simulink library "gm_TxLUT_RxCapture_4x4_HDL_IQ_lib"  (R2019b)
settings: Solver=VariableStepAuto  StartTime=0.0  StopTime=10.0  RelTol=1e-3
undefined symbols (not defined in the file or in its folder): AXI4, Lite
libraries: axiinterfacelib x11
settings Model: Creator=ajtro  LastModifiedBy=ajtro

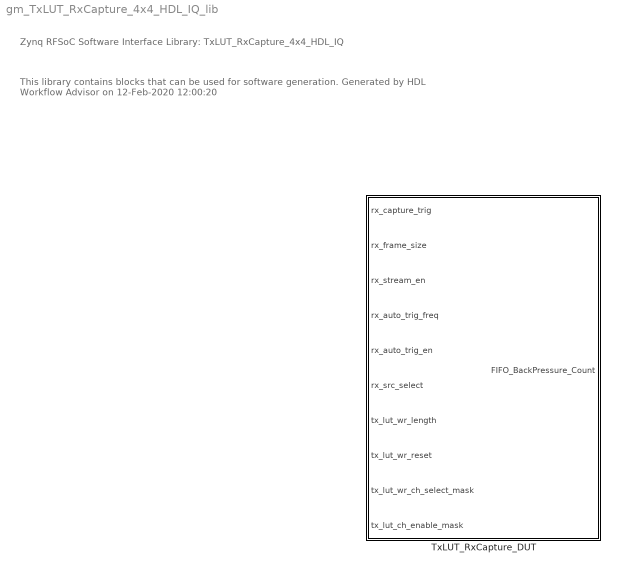
== system gm_TxLUT_RxCapture_4x4_HDL_IQ_lib ==
  note: Zynq RFSoC Software Interface Library: TxLUT_RxCapture_4x4_HDL_IQ
  note: This library contains blocks that can be used for software generation.
      |
      | Generated by HDL Workflow Advisor on 12-Feb-2020 12:00:20
  TxLUT_RxCapture_DUT : Subsystem  TreatAsAtomicUnit=on  mask(AXI4-Lite/AXI4 Interface){}
      mask help:
      | This is an automatically generated subsystem block.
      | This contains the AXI interface blocks that communicate with the DAC_ADC_HDL_Coder_IP IPCore generated from TxLUT_RxCapture_4x4_HDL_IQ/TxLUT_RxCapture_DUT subsystem.
      mask Display: disp(sprintf('Xilinx Zynq \nAXI Interface'));

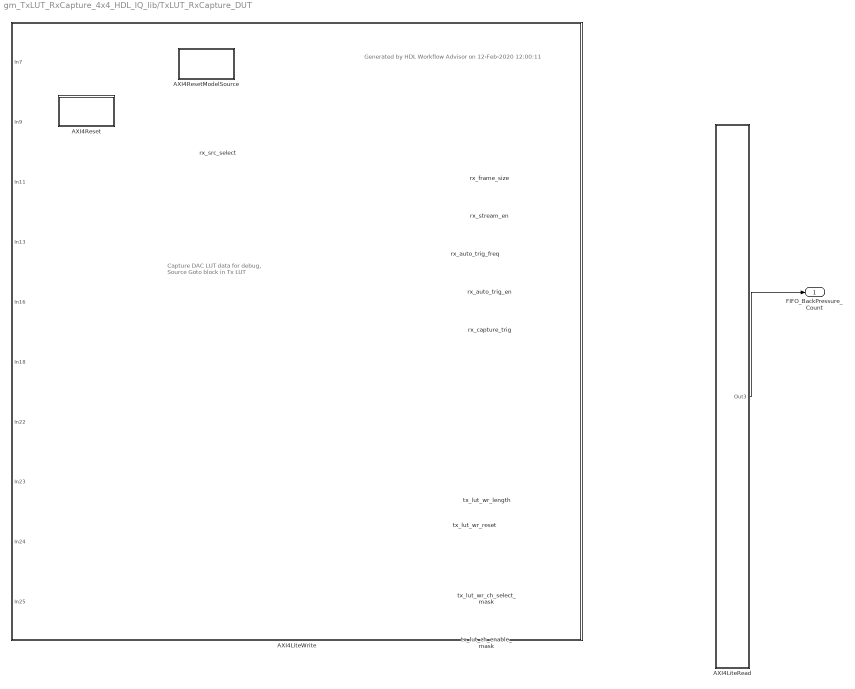
== system gm_TxLUT_RxCapture_4x4_HDL_IQ_lib/TxLUT_RxCapture_DUT ==
  note: Generated by HDL Workflow Advisor on 12-Feb-2020 12:00:11
  note: Capture DAC LUT data for debug,
      | Source Goto block in Tx LUT
  rx_capture_trig : Inport
  rx_frame_size : Inport  Port=2
  rx_stream_en : Inport  Port=3
  rx_auto_trig_freq : Inport  Port=4
  rx_auto_trig_en : Inport  Port=5
  rx_src_select : Inport  Port=6  OutDataTypeStr=fixdt(0,1,0)
  tx_lut_wr_length : Inport  Port=7
  tx_lut_wr_reset : Inport  Port=8
  tx_lut_wr_ch_select_mask : Inport  Port=9
  tx_lut_ch_enable_mask : Inport  Port=10
  AXI4LiteRead : Subsystem  Priority=10
  AXI4LiteWrite : Subsystem  Priority=1
  AXI4Reset : Subsystem  mask(System Start){ShowInLibBrowser=0}
      mask prompts: ShowInLibBrowser "Simulink:masks:CustCodeMaskParam1_MP"
      settings: CopyFcn=cccopyfcn(gcb)  OpenFcn=ccopenfcn('System Start Function')
      mask Help: eval('feval(''rtwprivate'',''rtwhelpview'',''rtw_sys_start_block'')');
      mask Display: disp('System\nStart');
  AXI4ResetModelSource : Subsystem  mask(Model Source){ShowInLibBrowser=0}
      mask prompts: ShowInLibBrowser "Simulink:masks:CustCodeMaskParam1_MP"
      settings: CopyFcn=cccopyfcn(gcb)  OpenFcn=ccopenfcn('Model Source')
      mask Help: eval('feval(''rtwprivate'',''rtwhelpview'',''rtw_model_source_block'')');
      mask Display: disp('Model\nSource');
  FIFO_BackPressure_Count : Outport  VectorParamsAs1DForOutWhenUnconnected=off
  wires:
  AXI4LiteRead/1(Out3) -> FIFO_BackPressure_Count/1
  tx_lut_ch_enable_mask/1 -> AXI4LiteWrite/10(In25)
  tx_lut_wr_ch_select_mask/1 -> AXI4LiteWrite/9(In24)
  tx_lut_wr_reset/1 -> AXI4LiteWrite/8(In23)
  tx_lut_wr_length/1 -> AXI4LiteWrite/7(In22)
  rx_capture_trig/1 -> AXI4LiteWrite/6(In18)
  rx_auto_trig_en/1 -> AXI4LiteWrite/5(In16)
  rx_auto_trig_freq/1 -> AXI4LiteWrite/4(In13)
  rx_stream_en/1 -> AXI4LiteWrite/3(In11)
  rx_frame_size/1 -> AXI4LiteWrite/2(In9)
  rx_src_select/1 -> AXI4LiteWrite/1(In7)

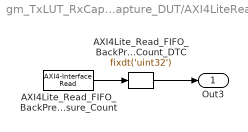
== system gm_TxLUT_RxCapture_4x4_HDL_IQ_lib/TxLUT_RxCapture_DUT/AXI4LiteRead ==
  AXI4Lite_Read_FIFO_BackPressure_Count : axiinterfacelib/AXI4-Interface Read  Priority=5  AXIInterfaceType=AXI4-Lite  DeviceName=/dev/mwipcore  RegisterOffset=hex2dec('134')  DataLength=1  DataType=uint32  SampleTime=-1  blockPlatform=ZYNQ  SimulateUsing=Interpreted Execution
      settings: SourceProductName=Embedded Coder Support Package for Xilinx Zynq Platform  SourceProductBaseCode=ECZYNQ7000
  AXI4Lite_Read_FIFO_BackPressure_Count_DTC : DataTypeConversion  OutDataTypeStr=fixdt('uint32')  ConvertRealWorld=Stored Integer (SI)
  Out3 : Outport
  wires:
  AXI4Lite_Read_FIFO_BackPressure_Count_DTC/1 -> Out3/1
  AXI4Lite_Read_FIFO_BackPressure_Count/1 -> AXI4Lite_Read_FIFO_BackPressure_Count_DTC/1

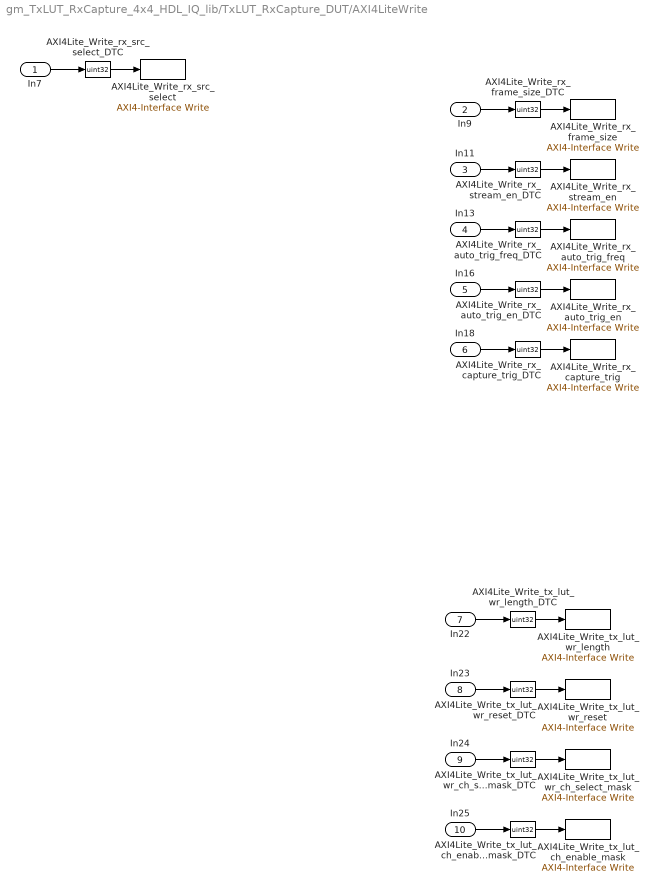
== system gm_TxLUT_RxCapture_4x4_HDL_IQ_lib/TxLUT_RxCapture_DUT/AXI4LiteWrite ==
  In7 : Inport
  In9 : Inport  Port=2
  In11 : Inport  Port=3
  In13 : Inport  Port=4
  In16 : Inport  Port=5
  In18 : Inport  Port=6
  In22 : Inport  Port=7
  In23 : Inport  Port=8
  In24 : Inport  Port=9
  In25 : Inport  Port=10
  AXI4Lite_Write_rx_auto_trig_en : axiinterfacelib/AXI4-Interface Write  Priority=20  AXIInterfaceType=AXI4-Lite  DeviceName=/dev/mwipcore  RegisterOffset=hex2dec('110')  blockPlatform=ZYNQ  SimulateUsing=Interpreted execution
      settings: SourceProductName=Embedded Coder Support Package for Xilinx Zynq Platform  SourceProductBaseCode=ECZYNQ7000
  AXI4Lite_Write_rx_auto_trig_en_DTC : DataTypeConversion  OutDataTypeStr=uint32  ConvertRealWorld=Stored Integer (SI)
  AXI4Lite_Write_rx_auto_trig_freq : axiinterfacelib/AXI4-Interface Write  Priority=19  AXIInterfaceType=AXI4-Lite  DeviceName=/dev/mwipcore  RegisterOffset=hex2dec('10C')  blockPlatform=ZYNQ  SimulateUsing=Interpreted execution
      settings: SourceProductName=Embedded Coder Support Package for Xilinx Zynq Platform  SourceProductBaseCode=ECZYNQ7000
  AXI4Lite_Write_rx_auto_trig_freq_DTC : DataTypeConversion  OutDataTypeStr=uint32  ConvertRealWorld=Stored Integer (SI)
  AXI4Lite_Write_rx_capture_trig : axiinterfacelib/AXI4-Interface Write  Priority=16  AXIInterfaceType=AXI4-Lite  DeviceName=/dev/mwipcore  RegisterOffset=hex2dec('100')  blockPlatform=ZYNQ  SimulateUsing=Interpreted execution
      settings: SourceProductName=Embedded Coder Support Package for Xilinx Zynq Platform  SourceProductBaseCode=ECZYNQ7000
  AXI4Lite_Write_rx_capture_trig_DTC : DataTypeConversion  OutDataTypeStr=uint32  ConvertRealWorld=Stored Integer (SI)
  AXI4Lite_Write_rx_frame_size : axiinterfacelib/AXI4-Interface Write  Priority=17  AXIInterfaceType=AXI4-Lite  DeviceName=/dev/mwipcore  RegisterOffset=hex2dec('104')  blockPlatform=ZYNQ  SimulateUsing=Interpreted execution
      settings: SourceProductName=Embedded Coder Support Package for Xilinx Zynq Platform  SourceProductBaseCode=ECZYNQ7000
  AXI4Lite_Write_rx_frame_size_DTC : DataTypeConversion  OutDataTypeStr=uint32  ConvertRealWorld=Stored Integer (SI)
  AXI4Lite_Write_rx_src_select : axiinterfacelib/AXI4-Interface Write  Priority=21  AXIInterfaceType=AXI4-Lite  DeviceName=/dev/mwipcore  RegisterOffset=hex2dec('114')  blockPlatform=ZYNQ  SimulateUsing=Interpreted execution
      settings: SourceProductName=Embedded Coder Support Package for Xilinx Zynq Platform  SourceProductBaseCode=ECZYNQ7000
  AXI4Lite_Write_rx_src_select_DTC : DataTypeConversion  OutDataTypeStr=uint32  ConvertRealWorld=Stored Integer (SI)
  AXI4Lite_Write_rx_stream_en : axiinterfacelib/AXI4-Interface Write  Priority=18  AXIInterfaceType=AXI4-Lite  DeviceName=/dev/mwipcore  RegisterOffset=hex2dec('108')  blockPlatform=ZYNQ  SimulateUsing=Interpreted execution
      settings: SourceProductName=Embedded Coder Support Package for Xilinx Zynq Platform  SourceProductBaseCode=ECZYNQ7000
  AXI4Lite_Write_rx_stream_en_DTC : DataTypeConversion  OutDataTypeStr=uint32  ConvertRealWorld=Stored Integer (SI)
  AXI4Lite_Write_tx_lut_ch_enable_mask : axiinterfacelib/AXI4-Interface Write  Priority=25  AXIInterfaceType=AXI4-Lite  DeviceName=/dev/mwipcore  RegisterOffset=hex2dec('124')  blockPlatform=ZYNQ  SimulateUsing=Interpreted execution
      settings: SourceProductName=Embedded Coder Support Package for Xilinx Zynq Platform  SourceProductBaseCode=ECZYNQ7000
  AXI4Lite_Write_tx_lut_ch_enable_mask_DTC : DataTypeConversion  OutDataTypeStr=uint32  ConvertRealWorld=Stored Integer (SI)
  AXI4Lite_Write_tx_lut_wr_ch_select_mask : axiinterfacelib/AXI4-Interface Write  Priority=24  AXIInterfaceType=AXI4-Lite  DeviceName=/dev/mwipcore  RegisterOffset=hex2dec('120')  blockPlatform=ZYNQ  SimulateUsing=Interpreted execution
      settings: SourceProductName=Embedded Coder Support Package for Xilinx Zynq Platform  SourceProductBaseCode=ECZYNQ7000
  AXI4Lite_Write_tx_lut_wr_ch_select_mask_DTC : DataTypeConversion  OutDataTypeStr=uint32  ConvertRealWorld=Stored Integer (SI)
  AXI4Lite_Write_tx_lut_wr_length : axiinterfacelib/AXI4-Interface Write  Priority=22  AXIInterfaceType=AXI4-Lite  DeviceName=/dev/mwipcore  RegisterOffset=hex2dec('118')  blockPlatform=ZYNQ  SimulateUsing=Interpreted execution
      settings: SourceProductName=Embedded Coder Support Package for Xilinx Zynq Platform  SourceProductBaseCode=ECZYNQ7000
  AXI4Lite_Write_tx_lut_wr_length_DTC : DataTypeConversion  OutDataTypeStr=uint32  ConvertRealWorld=Stored Integer (SI)
  AXI4Lite_Write_tx_lut_wr_reset : axiinterfacelib/AXI4-Interface Write  Priority=23  AXIInterfaceType=AXI4-Lite  DeviceName=/dev/mwipcore  RegisterOffset=hex2dec('11C')  blockPlatform=ZYNQ  SimulateUsing=Interpreted execution
      settings: SourceProductName=Embedded Coder Support Package for Xilinx Zynq Platform  SourceProductBaseCode=ECZYNQ7000
  AXI4Lite_Write_tx_lut_wr_reset_DTC : DataTypeConversion  OutDataTypeStr=uint32  ConvertRealWorld=Stored Integer (SI)
  wires:
  In13/1 -> AXI4Lite_Write_rx_auto_trig_freq_DTC/1
  In22/1 -> AXI4Lite_Write_tx_lut_wr_length_DTC/1
  In23/1 -> AXI4Lite_Write_tx_lut_wr_reset_DTC/1
  In18/1 -> AXI4Lite_Write_rx_capture_trig_DTC/1
  In9/1 -> AXI4Lite_Write_rx_frame_size_DTC/1
  In24/1 -> AXI4Lite_Write_tx_lut_wr_ch_select_mask_DTC/1
  In11/1 -> AXI4Lite_Write_rx_stream_en_DTC/1
  In7/1 -> AXI4Lite_Write_rx_src_select_DTC/1
  AXI4Lite_Write_rx_capture_trig_DTC/1 -> AXI4Lite_Write_rx_capture_trig/1
  AXI4Lite_Write_rx_auto_trig_en_DTC/1 -> AXI4Lite_Write_rx_auto_trig_en/1
  In25/1 -> AXI4Lite_Write_tx_lut_ch_enable_mask_DTC/1
  AXI4Lite_Write_rx_stream_en_DTC/1 -> AXI4Lite_Write_rx_stream_en/1
  AXI4Lite_Write_rx_frame_size_DTC/1 -> AXI4Lite_Write_rx_frame_size/1
  AXI4Lite_Write_tx_lut_ch_enable_mask_DTC/1 -> AXI4Lite_Write_tx_lut_ch_enable_mask/1
  AXI4Lite_Write_rx_src_select_DTC/1 -> AXI4Lite_Write_rx_src_select/1
  AXI4Lite_Write_tx_lut_wr_ch_select_mask_DTC/1 -> AXI4Lite_Write_tx_lut_wr_ch_select_mask/1
  AXI4Lite_Write_tx_lut_wr_length_DTC/1 -> AXI4Lite_Write_tx_lut_wr_length/1
  In16/1 -> AXI4Lite_Write_rx_auto_trig_en_DTC/1
  AXI4Lite_Write_tx_lut_wr_reset_DTC/1 -> AXI4Lite_Write_tx_lut_wr_reset/1
  AXI4Lite_Write_rx_auto_trig_freq_DTC/1 -> AXI4Lite_Write_rx_auto_trig_freq/1

== system gm_TxLUT_RxCapture_4x4_HDL_IQ_lib/TxLUT_RxCapture_DUT/AXI4Reset ==

== system gm_TxLUT_RxCapture_4x4_HDL_IQ_lib/TxLUT_RxCapture_DUT/AXI4ResetModelSource ==
